simulink model "RailP_DDsync"  (R2016b)
settings: configuration reference "CodeGenConfigSet" (kept outside this file)
values from neighbouring files (symbols this model uses):
  RailP_pLin_CUR = Calibration.Parameter    [init_RailP_DDsync.m]
  RailP_pLin_CURX = Calibration.Parameter    [init_RailP_DDsync.m]
  RailP_uSRCMax_C = Calibration.Parameter    [init_RailP_DDsync.m]
  RailP_uSRCMin_C = Calibration.Parameter    [init_RailP_DDsync.m]
settings Model: Creator=lenovo  LastModifiedBy=wangrui
settings ConfigSetRef: SourceLocation=Base Workspace

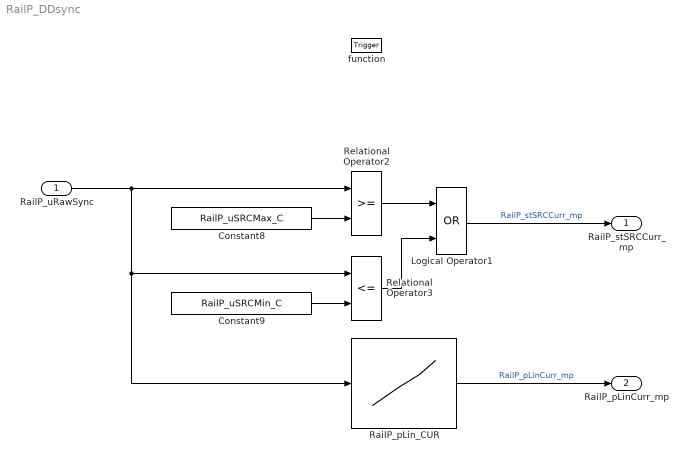
== system RailP_DDsync ==
  RailP_uRawSync : Inport  Tag=mv  Description=Raw value of rail pressure by teeth sample  OutMin=0  OutMax=5000  OutDataTypeStr=Ad_mv
  function : TriggerPort  TriggerType=function-call  VariantControl=Variant
  Constant8 : Constant  Value=RailP_uSRCMax_C
  Constant9 : Constant  Value=RailP_uSRCMin_C
  Logical Operator1 : Logic  Operator=OR  OutDataTypeStr=boolean
  RailP_pLin_CUR : Lookup_n-D  NumberOfTableDimensions=1  BreakpointsForDimension1=RailP_pLin_CURX  IndexSearchMethod=Linear search  BeginIndexSearchUsingPreviousIndexResult=on  UseOneInputPortForAllInputData=on  Table=RailP_pLin_CUR  ExtrapMethod=Clip  UseLastTableValue=on  InternalRulePriority=Speed  OutDataTypeStr=Inherit: Inherit via back propagation  SaturateOnIntegerOverflow=on
  Relational Operator2 : RelationalOperator  OutDataTypeStr=boolean  RndMeth=Nearest  InputSameDT=on
  Relational Operator3 : RelationalOperator  Operator=<=  OutDataTypeStr=boolean  RndMeth=Nearest  InputSameDT=on
  RailP_stSRCCurr_mp : Outport  Description=Maximum SRC default value  OutMin=0  OutMax=1  OutDataTypeStr=boolean
  RailP_pLinCurr_mp : Outport  Tag=bar  Description=Linearisation value current rail pressure  Port=2  OutMin=0  OutMax=2500  OutDataTypeStr=RailPressure_bar
  wires:
  Constant9/1 -> Relational Operator3/2
  Relational Operator2/1 -> Logical Operator1/1
  Relational Operator3/1 -> Logical Operator1/2
  Constant8/1 -> Relational Operator2/2
  Logical Operator1/1 -> RailP_stSRCCurr_mp/1  "RailP_stSRCCurr_mp"
  RailP_pLin_CUR/1 -> RailP_pLinCurr_mp/1  "RailP_pLinCurr_mp"
  RailP_uRawSync/1 -> RailP_pLin_CUR/1, Relational Operator3/1, Relational Operator2/1
